simulink model "Util"  (Simulink 7.5)
settings: Solver=ode45  StartTime=0.0  StopTime=10.0  RelTol=1e-3
settings Model: Creator=Joe P  LastModifiedBy=Joe P

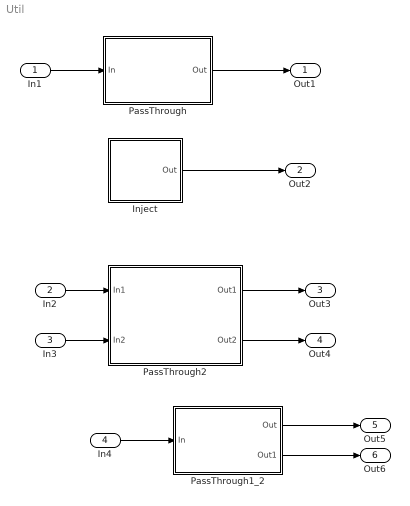
== system Util ==
  In1 : Inport  OutDataType=fixdt(1, 16)  OutScaling=2^0
  In2 : Inport  Port=2  OutDataType=fixdt(1, 16)  OutScaling=2^0
  In3 : Inport  Port=3  OutDataType=fixdt(1, 16)  OutScaling=2^0
  In4 : Inport  Port=4  OutDataType=fixdt(1, 16)  OutScaling=2^0
  Inject : Subsystem
  PassThrough : Subsystem
  PassThrough1_2 : Subsystem
  PassThrough2 : Subsystem
  Out1 : Outport  OutDataType=fixdt(1, 16)  OutScaling=2^0
  Out2 : Outport  Port=2  OutDataType=fixdt(1, 16)  OutScaling=2^0
  Out3 : Outport  Port=3  OutDataType=fixdt(1, 16)  OutScaling=2^0
  Out4 : Outport  Port=4  OutDataType=fixdt(1, 16)  OutScaling=2^0
  Out5 : Outport  Port=5  OutDataType=fixdt(1, 16)  OutScaling=2^0
  Out6 : Outport  Port=6  OutDataType=fixdt(1, 16)  OutScaling=2^0
  wires:
  In1/1 -> PassThrough/1(In)
  PassThrough/1(Out) -> Out1/1
  Inject/1(Out) -> Out2/1
  In2/1 -> PassThrough2/1(In1)
  PassThrough2/1(Out1) -> Out3/1
  In3/1 -> PassThrough2/2(In2)
  PassThrough2/2(Out2) -> Out4/1
  In4/1 -> PassThrough1_2/1(In)
  PassThrough1_2/1(Out) -> Out5/1
  PassThrough1_2/2(Out1) -> Out6/1

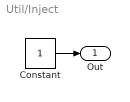
== system Util/Inject ==
  Constant : Constant  OutDataType=fixdt(1, 16)  OutScaling=2^0
  Out : Outport
  wires:
  Constant/1 -> Out/1

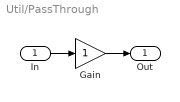
== system Util/PassThrough ==
  In : Inport
  Gain : Gain  ParameterDataType=fixdt(1, 16)  ParameterScaling=2^0  OutDataType=fixdt(1, 16)  OutScaling=2^0
  Out : Outport
  wires:
  In/1 -> Gain/1
  Gain/1 -> Out/1

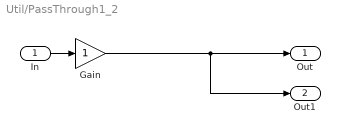
== system Util/PassThrough1_2 ==
  In : Inport
  Gain : Gain  ParameterDataType=fixdt(1, 16)  ParameterScaling=2^0  OutDataType=fixdt(1, 16)  OutScaling=2^0
  Out : Outport
  Out1 : Outport  Port=2
  wires:
  In/1 -> Gain/1
  Gain/1 -> Out/1, Out1/1

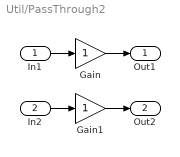
== system Util/PassThrough2 ==
  In1 : Inport
  In2 : Inport  Port=2
  Gain : Gain  ParameterDataType=fixdt(1, 16)  ParameterScaling=2^0  OutDataType=fixdt(1, 16)  OutScaling=2^0
  Gain1 : Gain  ParameterDataType=fixdt(1, 16)  ParameterScaling=2^0  OutDataType=fixdt(1, 16)  OutScaling=2^0
  Out1 : Outport
  Out2 : Outport  Port=2
  wires:
  In1/1 -> Gain/1
  Gain/1 -> Out1/1
  In2/1 -> Gain1/1
  Gain1/1 -> Out2/1
